simulink model "state_feedback_and_observer"  (R2017a)
settings: Solver=ode45  StartTime=0.0  StopTime=10.0  RelTol=1e-3  EnableMultiTasking=on
values from neighbouring files (symbols this model uses):
  k = acker(A,B,P)    [state_feedback_and_observer.m]    (also in state_feedback_and_observer2.m)
  L = acker(A',C',P1)    [state_feedback_and_observer.m]    (also in state_feedback_and_observer2.m)
settings Model: Creator=IVDL  LastModifiedBy=edward
settings DataIOCC: LimitDataPoints=on  SaveFormat=Array
settings OptimizationCC: LifeSpan=inf
settings DebuggingCC: UnderspecifiedInitializationDetection=Classic  MergeDetectMultiDrivingBlocksExec=none  SolverPrmCheckMsg=warning  StateNameClashWarn=warning  SFUnexpectedBacktrackingDiag=warning  SFNoUnconditionalDefaultTransitionDiag=warning  SFExecutionAtInitializationDiag=none
settings HardwareCC: ProdBitPerPointer=32  ProdBitPerSizeT=32  ProdBitPerPtrDiffT=32  ProdLargestAtomicFloat=None  ProdIntDivRoundTo=Undefined  ProdEndianess=Unspecified  ProdWordSize=32  ProdHWDeviceType=32-bit Generic
settings ModelReferenceCC: PropagateSignalLabelsOutOfModel=off
settings GRTTargetCC: TargetLangStandard=C89/C90 (ANSI)  GeneratePreprocessorConditionals=Disable all
settings ConfigComp: CovMetricSettings=dw  CovHtmlReporting=on  CovSaveCumulativeToWorkspaceVar=on  CovSaveSingleToWorkspaceVar=on  CovExternalEMLEnable=off

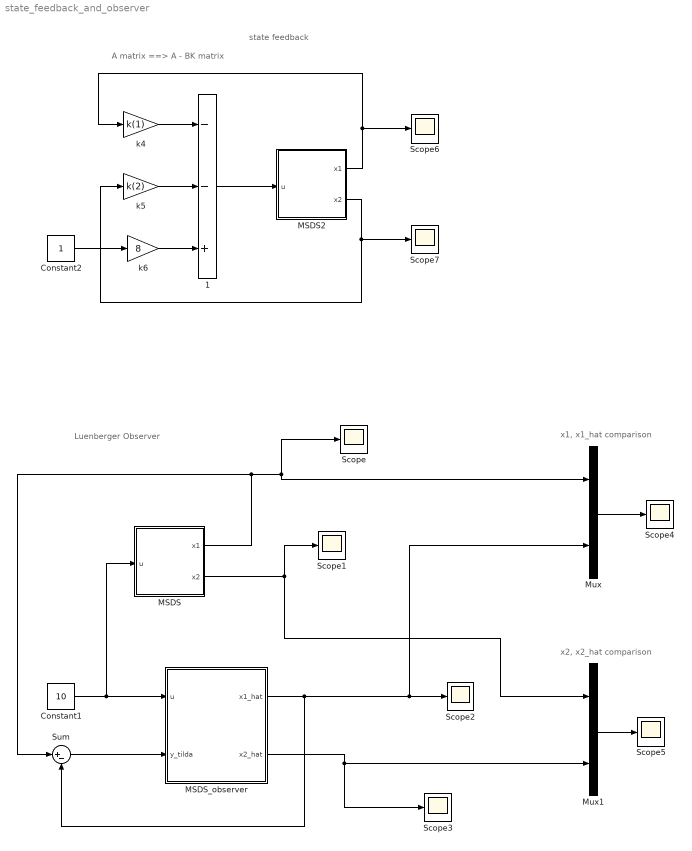
== system state_feedback_and_observer ==
  note: Luenberger Observer
  note: x1, x1_hat comparison
  note: x2, x2_hat comparison
  note: A matrix ==> A - BK matrix
  note: state feedback
  " 1" : Sum  Inputs=--+
  Constant1 : Constant  Value=10
  Constant2 : Constant
  MSDS : Subsystem
  MSDS2 : Subsystem
  MSDS_observer : Subsystem
  Mux : Mux  Inputs=2
  Mux1 : Mux  Inputs=2
  Scope{,1..7} (8 alike) : Scope
  Sum : Sum  Inputs=|+-
  k4 : Gain  Gain=k(1)
  k5 : Gain  Gain=k(2)
  k6 : Gain  Gain=8
  wires:
  MSDS/1(x1) -> Sum/1, Scope/1, Mux/1
  MSDS/2(x2) -> Scope1/1, Mux1/1
  MSDS_observer/1(x1_hat) -> Sum/2, Mux/2, Scope2/1
  Constant1/1 -> MSDS_observer/1(u), MSDS/1(u)
  Sum/1 -> MSDS_observer/2(y_tilda)
  MSDS_observer/2(x2_hat) -> Mux1/2, Scope3/1
  Mux/1 -> Scope4/1
  Mux1/1 -> Scope5/1
  MSDS2/1(x1) -> k4/1, Scope6/1
  MSDS2/2(x2) -> Scope7/1, k5/1
  k4/1 -> " 1"/1
  k5/1 -> " 1"/2
  Constant2/1 -> k6/1
  k6/1 -> " 1"/3
  " 1"/1 -> MSDS2/1(u)

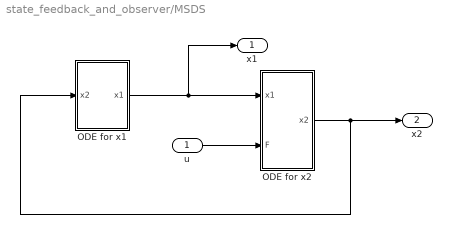
== system state_feedback_and_observer/MSDS ==
  u : Inport
  ODE for x1 : Subsystem
  ODE for x2 : Subsystem
  x1 : Outport
  x2 : Outport  Port=2
  wires:
  ODE for x2/1(x2) -> x2/1, ODE for x1/1(x2)
  u/1 -> ODE for x2/2(F)
  ODE for x1/1(x1) -> x1/1, ODE for x2/1("x1 ")

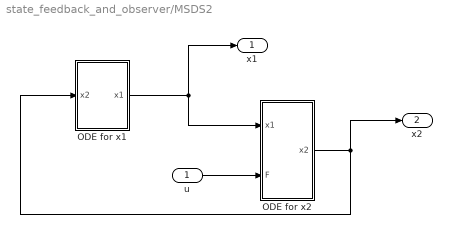
== system state_feedback_and_observer/MSDS2 ==
  u : Inport
  ODE for x1 : Subsystem
  ODE for x2 : Subsystem
  x1 : Outport
  x2 : Outport  Port=2
  wires:
  ODE for x2/1(x2) -> x2/1, ODE for x1/1(x2)
  u/1 -> ODE for x2/2(F)
  ODE for x1/1(x1) -> x1/1, ODE for x2/1("x1 ")

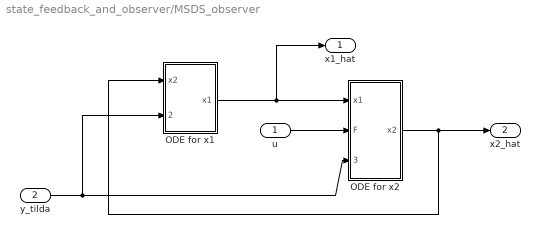
== system state_feedback_and_observer/MSDS_observer ==
  u : Inport
  y_tilda : Inport  Port=2
  ODE for x1 : Subsystem
  ODE for x2 : Subsystem
  x1_hat : Outport
  x2_hat : Outport  Port=2
  wires:
  ODE for x1/1(x1) -> x1_hat/1, ODE for x2/1("x1 ")
  u/1 -> ODE for x2/2(F)
  ODE for x2/1(x2) -> x2_hat/1, ODE for x1/1(x2)
  y_tilda/1 -> ODE for x2/3("y_tilda "), ODE for x1/2("y_tilda ")

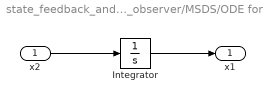
== system state_feedback_and_observer/MSDS/ODE for x1 ==
  x2 : Inport
  Integrator : Integrator
  x1 : Outport
  wires:
  Integrator/1 -> x1/1
  x2/1 -> Integrator/1

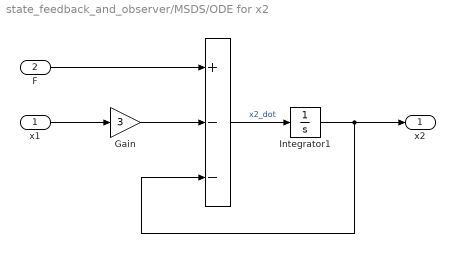
== system state_feedback_and_observer/MSDS/ODE for x2 ==
  "x1 " : Inport
  F : Inport  Port=2
  " " : Sum  Inputs=+--
  Gain : Gain  Gain=3
  Integrator1 : Integrator
  x2 : Outport
  wires:
  F/1 -> " "/1
  Integrator1/1 -> x2/1, " "/3
  Gain/1 -> " "/2
  " "/1 -> Integrator1/1  "x2_dot"
  "x1 "/1 -> Gain/1

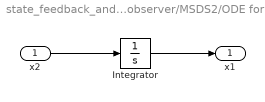
== system state_feedback_and_observer/MSDS2/ODE for x1 ==
  x2 : Inport
  Integrator : Integrator
  x1 : Outport
  wires:
  Integrator/1 -> x1/1
  x2/1 -> Integrator/1

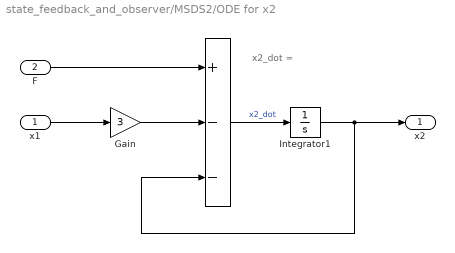
== system state_feedback_and_observer/MSDS2/ODE for x2 ==
  note: x2_dot =
  "x1 " : Inport
  F : Inport  Port=2
  " " : Sum  Inputs=+--
  Gain : Gain  Gain=3
  Integrator1 : Integrator
  x2 : Outport
  wires:
  F/1 -> " "/1
  Integrator1/1 -> x2/1, " "/3
  Gain/1 -> " "/2
  " "/1 -> Integrator1/1  "x2_dot"
  "x1 "/1 -> Gain/1

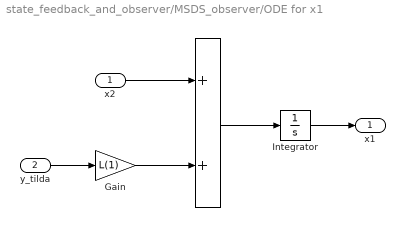
== system state_feedback_and_observer/MSDS_observer/ODE for x1 ==
  x2 : Inport
  "y_tilda " : Inport  Port=2
  " " : Sum
  Gain : Gain  Gain=L(1)
  Integrator : Integrator
  x1 : Outport
  wires:
  Integrator/1 -> x1/1
  x2/1 -> " "/1
  Gain/1 -> " "/2
  "y_tilda "/1 -> Gain/1
  " "/1 -> Integrator/1

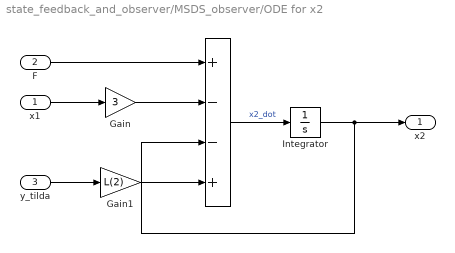
== system state_feedback_and_observer/MSDS_observer/ODE for x2 ==
  "x1 " : Inport
  F : Inport  Port=2
  "y_tilda " : Inport  Port=3
  " " : Sum  Inputs=+--+
  Gain : Gain  Gain=3
  Gain1 : Gain  Gain=L(2)
  Integrator : Integrator
  x2 : Outport
  wires:
  "x1 "/1 -> Gain/1
  " "/1 -> Integrator/1  "x2_dot"
  Gain/1 -> " "/2
  Integrator/1 -> " "/3, x2/1
  F/1 -> " "/1
  Gain1/1 -> " "/4
  "y_tilda "/1 -> Gain1/1
